simulink model "my_mass"  (R2021b)
settings: Solver=FixedStepAuto  StartTime=0.0  StopTime=10.0  RelTol=1e-3
settings Model: Creator=lywan  LastModifiedBy=lywan
settings RTWCC: GenCodeOnly=on  Toolchain=AUTOSAR Adaptive | CMake  TargetLang=C++
settings GRTTargetCC: TargetLangStandard=C++11 (ISO)

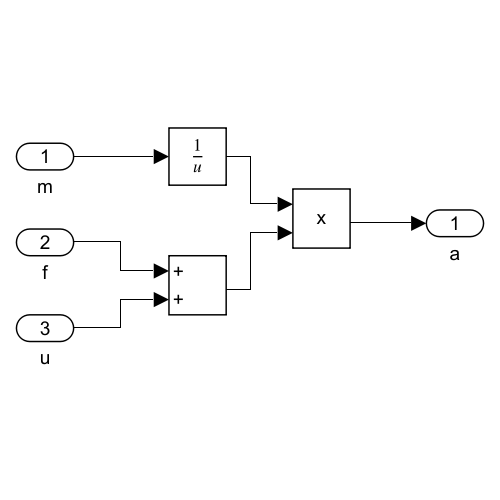
[thumbnail: Simulink's stored preview of the top-level diagram]
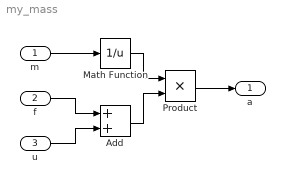
== system my_mass ==
  m : Inport
  f : Inport  Port=2
  u : Inport  Port=3
  Add : Sum
  Math Function : Math  Operator=reciprocal  SignedPower=on  RndMeth=Zero  SaturateOnIntegerOverflow=on
  Product : Product
  a : Outport
  wires:
  f/1 -> Add/1
  u/1 -> Add/2
  m/1 -> Math Function/1
  Product/1 -> a/1
  Math Function/1 -> Product/1
  Add/1 -> Product/2
